simulink model "mdaqdemo_pilbuf"  (R2013a)
settings: Solver=FixedStepDiscrete  StartTime=0.0  StopTime=inf  RelTol=1e-3
libraries: simulink x2
settings Model: Creator=peselnikmg  LastModifiedBy=skibool
settings DataIOCC: LimitDataPoints=off  SignalLoggingSaveFormat=ModelDataLogs  SaveOutput=off  SignalLogging=off  DSMLogging=off  SaveTime=off
settings OptimizationCC: InlineParams=on  OptimizeModelRefInitCode=on  LifeSpan=1
settings HardwareCC: ProdBitPerLong=40  ProdLargestAtomicInteger=Integer  ProdIntDivRoundTo=Zero  ProdEndianess=LittleEndian  ProdHWDeviceType=Texas Instruments->C6000
settings RTWCC: SystemTargetFile=microdaq.tlc  TemplateMakefile=microdaq.tmf  PostCodeGenCommand=microdaq_postcodegen(buildInfo)  Description=MicroDAQ Real-Time Measurement System  ProcessScript=microdaq_make_rtw_hook
settings CodeAppCC: IgnoreCustomStorageClasses=off
settings STFCustomTargetCC: CodeReplacementLibrary=TI C674x  CombineOutputUpdateFcns=on  ERTCustomFileBanners=on  SupportContinuousTime=off  SupportNonInlinedSFcns=off  MATLABClassNameForMDSCustomization=Simulink.SoftwareTarget.ERTCustomization  SystemTargetFile=microdaq.tlc
settings ERTTargetCC: CodeReplacementLibrary=TI C674x  GenerateSampleERTMain=off  ParMdlRefBuildCompliant=off  CompOptLevelCompliant=off  ConcurrentExecutionCompliant=off  ERTFirstTimeCompliant=off  ModelStepFunctionPrototypeControlCompliant=off  CPPClassGenCompliant=off  ERTCustomFileTemplate=microdaq_main.tlc

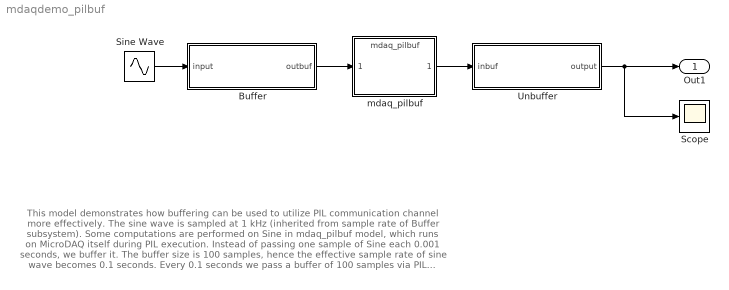
== system mdaqdemo_pilbuf ==
  note: This model demonstrates how buffering can be used to utilize PIL
      | communication channel more effectively.
      |
      | The sine wave is sampled at 1 kHz (inherited from sample rate of Buffer subsystem).
      | Some computations are performed on Sine in mdaq_pilbuf model, which
      | runs on MicroDAQ itself during PIL execution.
      |
      | Instead of passing one sample of Sine each 0.001 seconds, we buffer it.
      | The buffer size is 100 samples, hence the effective sample rate of sine wave
      | becomes 0.1 seconds. Every 0.1 seconds we pass a buffer of 100 samples via
      | PIL interface instead of passing 1 sample each 0.001 seconds.
      |
      | Colors in the model denote different sample rates. Press Ctrl+J to show the legend.
      |
      | After computations have been carried out with our buffered Sine, we pass it back
      | to Simulink as a buffer. We then unbuffer the signal to visualize it.
  Buffer : Subsystem  TreatAsAtomicUnit=on  mask{BufSize=100, Ts=0.001}
      mask prompts: BufSize "Buffer Size:"; Ts "Sample Time:"
      mask Display:
      | fprintf('Buffer Size: %d\n\n', BufSize);
      | fprintf('\n\nSample Time: %g\n', Ts);
  Scope : Scope
      settings: YMin=155  YMax=165  MaxDataPoints=10000
  Sine Wave : Sin
  Unbuffer : Subsystem  TreatAsAtomicUnit=on  mask{BufSize=100, Ts=0.001}
      mask prompts: BufSize "Buffer Size:"; Ts "Sample Time:"
      mask Display:
      | fprintf('Buffer Size: %d\n\n', BufSize);
      | fprintf('\n\nSample Time: %g\n', Ts);
  mdaq_pilbuf : ModelReference  ModelNameDialog=mdaq_pilbuf  SimulationMode=Processor-in-the-loop (PIL)  ModelReferenceVersion=1.29  CopyOfModelName=mdaq_pilbuf  DefaultDataLogging=on
  Out1 : Outport
  wires:
  Sine Wave/1 -> Buffer/1(input)
  Unbuffer/1(output) -> Scope/1, Out1/1
  Buffer/1(outbuf) -> mdaq_pilbuf/1
  mdaq_pilbuf/1 -> Unbuffer/1(inbuf)

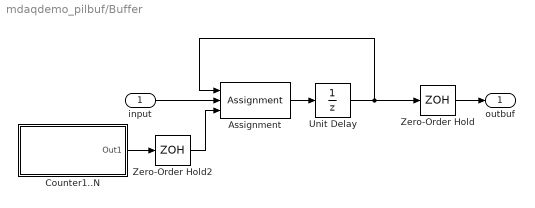
== system mdaqdemo_pilbuf/Buffer ==
  input : Inport  SampleTime=Ts
  Assignment : Assignment  IndexOptions=Index vector (port)  Indices=1  OutputSizes=100
  Counter1..N : Subsystem
      mask Display: disp('Counter')
  Unit Delay : UnitDelay  InitialCondition=zeros(BufSize,1)  SampleTime=Ts
  Zero-Order Hold : ZeroOrderHold  SampleTime=BufSize*Ts
  Zero-Order Hold2 : ZeroOrderHold  SampleTime=Ts
  outbuf : Outport
  wires:
  input/1 -> Assignment/2
  Zero-Order Hold2/1 -> Assignment/3
  Assignment/1 -> Unit Delay/1
  Zero-Order Hold/1 -> outbuf/1
  Counter1..N/1(Out1) -> Zero-Order Hold2/1
  Unit Delay/1 -> Assignment/1, Zero-Order Hold/1

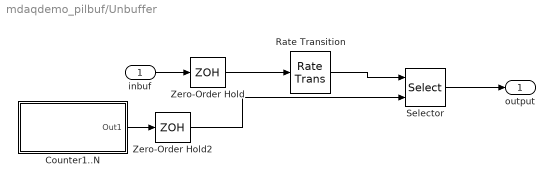
== system mdaqdemo_pilbuf/Unbuffer ==
  inbuf : Inport  SampleTime=Ts
  Counter1..N : Subsystem
      mask Display: disp('Counter')
  Rate Transition : RateTransition
  Selector : Selector  InputPortWidth=BufSize  IndexOptions=Index vector (port)  Indices=[1 3]  OutputSizes=1
  Zero-Order Hold : ZeroOrderHold  SampleTime=BufSize*Ts
  Zero-Order Hold2 : ZeroOrderHold  SampleTime=Ts
  output : Outport
  wires:
  Counter1..N/1(Out1) -> Zero-Order Hold2/1
  Zero-Order Hold2/1 -> Selector/2
  inbuf/1 -> Zero-Order Hold/1
  Selector/1 -> output/1
  Zero-Order Hold/1 -> Rate Transition/1
  Rate Transition/1 -> Selector/1

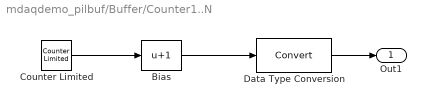
== system mdaqdemo_pilbuf/Buffer/Counter1..N ==
  Bias : Bias  Bias=1
  Counter Limited : simulink/Sources/Counter Limited  uplimit=BufSize-1  tsamp=-1
  Data Type Conversion : DataTypeConversion
  Out1 : Outport
  wires:
  Counter Limited/1 -> Bias/1
  Bias/1 -> Data Type Conversion/1
  Data Type Conversion/1 -> Out1/1

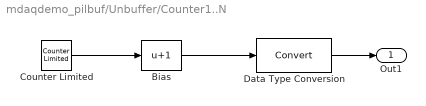
== system mdaqdemo_pilbuf/Unbuffer/Counter1..N ==
  Bias : Bias  Bias=1
  Counter Limited : simulink/Sources/Counter Limited  uplimit=BufSize-1  tsamp=-1
  Data Type Conversion : DataTypeConversion
  Out1 : Outport
  wires:
  Data Type Conversion/1 -> Out1/1
  Bias/1 -> Data Type Conversion/1
  Counter Limited/1 -> Bias/1
